simulink model "incalzire_pardoseala"  (R2024a)
settings: Solver=VariableStepAuto  StartTime=0.0  StopTime=12000  RelTol=1e-3
values from neighbouring files (symbols this model uses):
  A = [-1/Tp 1/Tp; kp/(kc*Tc) (-1)*(1+kp/kc)/Tc]    [parametrii.m]
  B = [kE/(kp*Tp) 0; 0 1/Tc]    [parametrii.m]
  C = eye(2)    [parametrii.m]
  D = zeros(2)    [parametrii.m]
  kc = 125    [parametrii.m]
  kE = 1000    [parametrii.m]
  kp = 500    [parametrii.m]
  Tc = 300    [parametrii.m]
  Tp = 60    [parametrii.m]
settings Model: Creator=paulhondola  LastModifiedBy=paulhondola

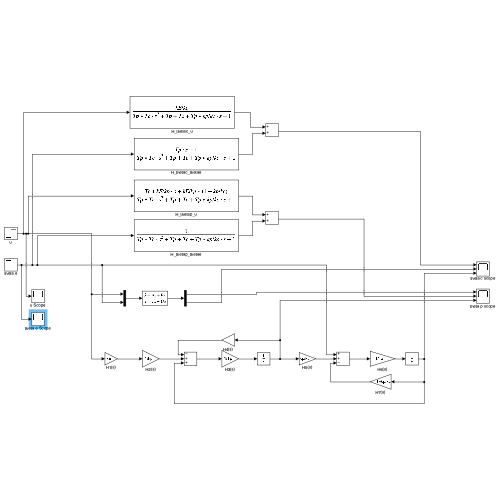
[thumbnail: Simulink's stored preview of the top-level diagram]
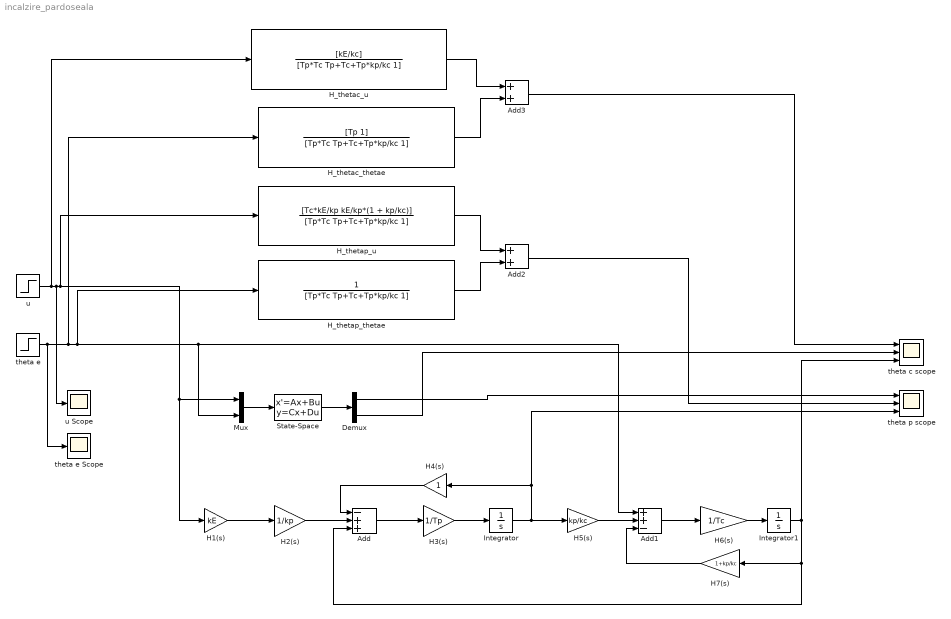
== system incalzire_pardoseala ==
  Add : Sum  Inputs=-++
  Add1 : Sum  Inputs=++-
  Add2 : Sum
  Add3 : Sum
  Demux : Demux  Outputs=2
  H1(s) : Gain  Gain=kE
  H2(s) : Gain  Gain=1/kp
  H3(s) : Gain  Gain=1/Tp
  H4(s) : Gain
  H5(s) : Gain  Gain=kp/kc
  H6(s) : Gain  Gain=1/Tc
  H7(s) : Gain  Gain=1+kp/kc
  H_thetac_thetae : TransferFcn  Numerator=[Tp 1]  Denominator=[Tp*Tc Tp+Tc+Tp*kp/kc 1]
  H_thetac_u : TransferFcn  Numerator=[kE/kc]  Denominator=[Tp*Tc Tp+Tc+Tp*kp/kc 1]
  H_thetap_thetae : TransferFcn  Denominator=[Tp*Tc Tp+Tc+Tp*kp/kc 1]
  H_thetap_u : TransferFcn  Numerator=[Tc*kE/kp kE/kp*(1 + kp/kc)]  Denominator=[Tp*Tc Tp+Tc+Tp*kp/kc 1]
  Integrator : Integrator
  Integrator1 : Integrator
  Mux : Mux  Inputs=2
  State-Space : StateSpace  A=A  B=B  C=C  D=D  InitialCondition=0
  theta c scope : Scope  NumInputPorts=3
  theta e : Step  Time=5000  After=-10  SampleTime=0
  theta e Scope : Scope
  theta p scope : Scope  NumInputPorts=3
  u : Step  Time=0  After=2.5  SampleTime=0
  u Scope : Scope
  wires:
  Mux/1 -> State-Space/1
  State-Space/1 -> Demux/1
  u/1 -> H_thetac_u/1, u Scope/1, H_thetap_u/1, H1(s)/1, Mux/1
  theta e/1 -> H_thetac_thetae/1, H_thetap_thetae/1, Add1/1, Mux/2, theta e Scope/1
  H1(s)/1 -> H2(s)/1
  H2(s)/1 -> Add/2
  Add/1 -> H3(s)/1
  H3(s)/1 -> Integrator/1
  Integrator/1 -> H5(s)/1, theta p scope/3, H4(s)/1
  H4(s)/1 -> Add/1
  H5(s)/1 -> Add1/2
  H6(s)/1 -> Integrator1/1
  Add1/1 -> H6(s)/1
  Integrator1/1 -> theta c scope/3, Add/3, H7(s)/1
  H7(s)/1 -> Add1/3
  H_thetac_u/1 -> Add3/1
  H_thetac_thetae/1 -> Add3/2
  H_thetap_u/1 -> Add2/1
  H_thetap_thetae/1 -> Add2/2
  Add3/1 -> theta c scope/1
  Add2/1 -> theta p scope/2
  Demux/1 -> theta p scope/1
  Demux/2 -> theta c scope/2
